simulink subsystem "VDBSCAN"  (R2022b)
settings: Solver=VariableStepAuto  StartTime=0.0  StopTime=10.0  RelTol=1e-3
settings Model: Creator=smryk  LastModifiedBy=sathu

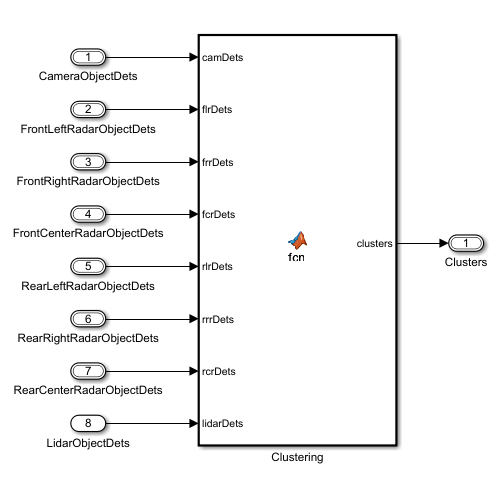
[thumbnail: Simulink's stored preview of the top-level diagram]
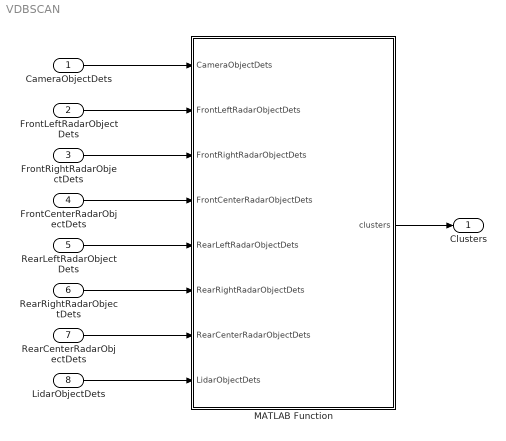
== system VDBSCAN ==
  CameraObjectDets : Inport  OutDataTypeStr=Bus: BusObjectDetections1
  FrontLeftRadarObjectDets : Inport  Port=2  OutDataTypeStr=Bus: BusDrivingRadarDataGenerator1
  FrontRightRadarObjectDets : Inport  Port=3  OutDataTypeStr=Bus: BusDrivingRadarDataGenerator1
  FrontCenterRadarObjectDets : Inport  Port=4  OutDataTypeStr=Bus: BusDrivingRadarDataGenerator1
  RearLeftRadarObjectDets : Inport  Port=5  OutDataTypeStr=Bus: BusDrivingRadarDataGenerator1
  RearRightRadarObjectDets : Inport  Port=6  OutDataTypeStr=Bus: BusDrivingRadarDataGenerator1
  RearCenterRadarObjectDets : Inport  Port=7  OutDataTypeStr=Bus: BusDrivingRadarDataGenerator1
  LidarObjectDets : Inport  Port=8
  MATLAB Function : MATLAB Function  TreatAsAtomicUnit=on
  Clusters : Outport  OutDataTypeStr=Bus: BusObjectDetections1
  wires:
  LidarObjectDets/1 -> MATLAB Function/8(LidarObjectDets)
  RearCenterRadarObjectDets/1 -> MATLAB Function/7(RearCenterRadarObjectDets)
  RearRightRadarObjectDets/1 -> MATLAB Function/6(RearRightRadarObjectDets)
  RearLeftRadarObjectDets/1 -> MATLAB Function/5(RearLeftRadarObjectDets)
  FrontCenterRadarObjectDets/1 -> MATLAB Function/4(FrontCenterRadarObjectDets)
  FrontRightRadarObjectDets/1 -> MATLAB Function/3(FrontRightRadarObjectDets)
  FrontLeftRadarObjectDets/1 -> MATLAB Function/2(FrontLeftRadarObjectDets)
  MATLAB Function/1(clusters) -> Clusters/1
  CameraObjectDets/1 -> MATLAB Function/1(CameraObjectDets)

== matlab function VDBSCAN/MATLAB Function ==
  data: CameraObjectDets input; clusters output Bus: BusObjectDetections1; FrontLeftRadarObjectDets input; FrontRightRadarObjectDets input; FrontCenterRadarObjectDets input; RearLeftRadarObjectDets input; RearRightRadarObjectDets input; RearCenterRadarObjectDets input; LidarObjectDets input
function clusters = fcn(CameraObjectDets, FrontLeftRadarObjectDets, FrontRightRadarObjectDets, FrontCenterRadarObjectDets, RearLeftRadarObjectDets, RearRightRadarObjectDets, RearCenterRadarObjectDets, LidarObjectDets)
    %clusters.Detections.Measurements(1)= xPos
    %clusters.Detections.Measurements(2)= yPos
    %clusters.NumDetections = number of clusters

    %format the data from the sensors
    sensorsData = formatSensorData(CameraObjectDets, FrontLeftRadarObjectDets, FrontRightRadarObjectDets, FrontCenterRadarObjectDets, RearLeftRadarObjectDets, RearRightRadarObjectDets, RearCenterRadarObjectDets, LidarObjectDets);
    
    k = 5; %NOTE: K can be adjusted 
    minPoints = k - 1; %minus one because k used in calculating epsilon has the points itself included as neighbouring points
    minDetections = 3; %minimum number of detections to validate a cluster

    epsilon = kNeighbours(sensorsData, k);

    %run DBSCAN
    allClusters = [0 0 0];
    for j = 1:size(epsilon, 1)
        idx = DBSCAN(epsilon(j), minPoints, sensorsData);

        clusterData = sensorsData(idx ~= -1, :);
        sensorsData = sensorsData(idx == -1, :);
        
        %Get the tracks 
        validIdx = idx(idx ~= -1);
        clusterNum = unique(validIdx);

        for m = 1:size(clusterNum,1)
            cluster = clusterData(validIdx == m, :);
            if (size(cluster,1) >= minDetections)
                centroid = mean(cluster);
                tracks = [centroid(1) centroid(2) size(cluster,1)];

                allClusters = [allClusters; tracks];
            end
        end  
    end
     
    finalClusters = allClusters(2:end,:); %strip off the first element since that was just a place hold for the size allTracks
    %finalClusters = [xPos yPos numDetections]

    measurements = zeros(50, 2);
    for j = 1:size(finalClusters, 1)
        measurements(j,:) = finalClusters(j,1:2);
    end
    

    clusters.NumDetections = size(finalClusters, 1);
    clusters.IsValidTime = boolean(0);
    
    fakeMeasurementParams.Frame = drivingCoordinateFrameType(0);
    fakeMeasurementParams.OriginPosition = [0; 0; 0];
    fakeMeasurementParams.Orientation = [0 0 0; 0 0 0; 0 0 0];
    fakeMeasurementParams.HasVelocity = boolean(0);
    
    fakeObjAttributes.TargetIndex = 0;

    for i = 1:50
        fakeDetection.Time = 0;
        fakeDetection.Measurement = [measurements(i,1); measurements(i,2); 0; 0; 0; 0];
        fakeDetection.MeasurementNoise = [0 0 0 0 0 0; 0 0 0 0 0 0; 0 0 0 0 0 0; 0 0 0 0 0 0; 0 0 0 0 0 0; 0 0 0 0 0 0];
        fakeDetection.SensorIndex = 0;
        fakeDetection.ObjectClassID = 0;
        fakeDetection.MeasurementParameters = fakeMeasurementParams;
        fakeDetection.ObjectAttributes = fakeObjAttributes;

        clusters.Detections(i) = fakeDetection;
    end
end 

function sensorsData = formatSensorData(CameraObjectDets, FrontLeftRadarObjectDets, FrontRightRadarObjectDets, FrontCenterRadarObjectDets, RearLeftRadarObjectDets, RearRightRadarObjectDets, RearCenterRadarObjectDets, LidarObjectDets)
    %% Format Sensor Data
    numFrontCamDets = CameraObjectDets.NumDetections;
    frontCamDetsArray = CameraObjectDets.Detections;
    
    numFrontLeftRadarDets = FrontLeftRadarObjectDets.NumDetections;
    frontLeftRadarDetsArray = FrontLeftRadarObjectDets.Detections;
    
    numFrontRightRadarDets = FrontRightRadarObjectDets.NumDetections;
    frontRightRadarDetsArray = FrontRightRadarObjectDets.Detections;


    numFrontCenterRadarDets = FrontCenterRadarObjectDets.NumDetections;
    frontCenterRadarDetsArray = FrontCenterRadarObjectDets.Detections;

    numRearLeftRadarDets = RearLeftRadarObjectDets.NumDetections;
    rearLeftRadarDetsArray = RearLeftRadarObjectDets.Detections;
    
    numRearRightRadarDets = RearRightRadarObjectDets.NumDetections;
    rearRightRadarDetsArray = RearRightRadarObjectDets.Detections;

    numRearCenterRadarDets = RearCenterRadarObjectDets.NumDetections;
    rearCenterRadarDetsArray = RearCenterRadarObjectDets.Detections;

    numLidarDets = LidarObjectDets.NumDetections;
    lidarObjectDetsArray = LidarObjectDets.Detections;
    
    %Get Front camera data [xPos, yPos]
    frontCamera = zeros(numFrontCamDets,2);
    for i = 1:numFrontCamDets
        detection = frontCamDetsArray(i);
        disp("Camera")
        disp(detection.MeasurementNoise)
        detectionState = detection.Measurement; 
        frontCamera(i,:)=[detectionState(1), detectionState(2)];
    end

    %Get front left radar data [xPos, yPos]
    frontLeftRadar = zeros(numFrontLeftRadarDets,2);
    for i = 1:numFrontLeftRadarDets
        detection = frontLeftRadarDetsArray(i);
        disp("Radar")
        disp(detection.MeasurementNoise)
        detectionState = detection.Measurement; 
        frontLeftRadar(i,:) = [detectionState(1), detectionState(2)];
    end

    %Get front right radar data [xPos, yPos]
    frontRightRadar = zeros(numFrontRightRadarDets, 2);
    for i = 1:numFrontRightRadarDets
        detection = frontRightRadarDetsArray(i);
        detectionState = detection.Measurement; 
        frontRightRadar(i,:) = [detectionState(1), detectionState(2)];
    end

    %Get front center radar data [xPos, yPos]
    frontCenterRadar = zeros(numFrontCenterRadarDets, 2);
    for i = 1:numFrontCenterRadarDets
        detection = frontCenterRadarDetsArray(i);
        detectionState = detection.Measurement; 
        frontCenterRadar(i,:) = [detectionState(1), detectionState(2)];
    end

    %Get rear left radar data [xPos, yPos]
    rearLeftRadar = zeros(numRearLeftRadarDets,2);
    for i = 1:numRearLeftRadarDets
        detection = rearLeftRadarDetsArray(i);
        detectionState = detection.Measurement; 
        rearLeftRadar(i,:) = [detectionState(1), detectionState(2)];
    end

    %Get rear right radar data [xPos, yPos]
    rearRightRadar = zeros(numRearRightRadarDets, 2);
    for i = 1:numRearRightRadarDets
        detection = rearRightRadarDetsArray(i);
        detectionState = detection.Measurement; 
        rearRightRadar(i,:) = [detectionState(1), detectionState(2)];
    end

    %Get rear center radar data [xPos, yPos]
    rearCenterRadar = zeros(numRearCenterRadarDets, 2);
    for i = 1:numRearCenterRadarDets
        detection = rearCenterRadarDetsArray(i);
        detectionState = detection.Measurement; 
        rearCenterRadar(i,:) = [detectionState(1), detectionState(2)];
    end

    %Get lidar data [xPos, yPos]
    lidar = zeros(numLidarDets,2);
    for i = 1:numLidarDets
        detection = lidarObjectDetsArray(i);
        detectionState = detection.Measurement; 
        lidar(i,:)=[detectionState(1), detectionState(2)];
    end

    %combine sensors' data into one matrix 
    sensorsData = [frontCamera; frontLeftRadar; frontRightRadar; frontCenterRadar; rearLeftRadar; rearRightRadar; rearCenterRadar; lidar];
end

function epsilon = kNeighbours(sensorsData, k)
    %INPUT
    %sensorsData = [xPos yPos]
    %k = int
    %OUTPUT
    %epsilon = [radius]
  
    kPoints = zeros(size(sensorsData,1),1);
    %find the kth nearest neighbour of all data points
    for i = 1:size(sensorsData, 1)
        currentPoint = sensorsData(i,:);
        distance = sqrt((sensorsData(:,1) - currentPoint(1)).^2 + (sensorsData(:,2) - currentPoint(2)).^2);
        sortedDistance = sort(distance);
        kPoints(i) = sortedDistance(k);
    end

    kPoints = sort(kPoints);
    [~, similarPoints] = ischange(kPoints);
    epsilon = unique(similarPoints);
    epsilon = epsilon(epsilon <= 1.5); %only allow epsilons less than 1.5

end

function clusters = DBSCAN(radius, minPoints, sensorsData)
    %% Algorithm- DBSCAN
    %INPUT
    %radius = int
    %minPoints = int
    %sensorsData = [xPos yPos] 
    %OUTPUT
    %clusters = [clusterNum] 
    
    %Find Core Points
    dataDim = size(sensorsData, 1);
    pointTypeData = [sensorsData zeros(dataDim,1)]; %[xPos yPos isCorePoint]

    for i = 1: dataDim
        pointTypeData(i,3) = findCorePoint(sensorsData(i,:), sensorsData, radius, minPoints);
    end

    %Organize the Corepoints into clusters
    corePointClusters = groupCorePoints(pointTypeData, radius);

    %Classify border points into the clusters
    clusterData = classifyBorderPoints(pointTypeData, corePointClusters, radius);

    clusters = clusterData(:,4);
end

%Determines if a point is a Core Point
function isCorePoint = findCorePoint (currentPoint, sensorData, radius, minPoints)
    %INPUT
    % currentPoint = [xPos yPos]
    %sensorData = [xPos yPos]
    %radius = float
    %minPoint = int
    %OUTPUT
    %isCorePoint = Boolean

    %find the relative distance of all points in the Data to the current point
    relativeDistance = sqrt((sensorData(:,1) - currentPoint(1)).^2 + (sensorData(:,2) - currentPoint(2)).^2);

    %Check if the number of neghboring points is less than minPoints
    counter = 0;
    for i = 1:size(sensorData,1)
        if (relativeDistance(i) <= radius)
            counter = counter + 1;
            if (counter >= minPoints)
                isCorePoint = true;
                return;
            end
        end
    end
    isCorePoint = false;
end

%Group core points into clusters
function corePointClusters = groupCorePoints(pointTypeData, radius)
    %INPUT
    %pointTypeData = [Boolean]
    %radius = float 
    %OUTPUT
    %corePointClusters = [xPos yPos isCorePoint clusterNum]
    
    corePointClusters = [pointTypeData ones(size(pointTypeData,1),1).*-1 ]; %[xPos yPos isCorePoint clusterNum]
    corePointData = [pointTypeData(pointTypeData(:,3) == 1, 1:2) find(pointTypeData(:,3) == 1)]; %[xPos yPos index] for Core Points in corePointCluster, index refers to location of point in corePointCluster
    cluster = []; %[xPos, yPos, clusterNum]
    clusterNumber = 1;

    while size(corePointData, 1) ~= 0
        %Takes whatever is first in corePointData as starting point for cluster
        cluster = [corePointData(1,1:2) clusterNumber]; %[xPos yPos clusterNum]
        
        %update the status of that point to the current cluster num
        corePointClusters(corePointData(1,3),4) = clusterNumber;

        corePointData = corePointData(2:end, :); %remove the point from the dataset so we don't have duplicates
        counter = 1;

        while counter <= size(cluster,1)
            %Use the position counter of cluster as a pointer to compare neighbouring core points
            %Use the first two columns of cluster as it contains the xPos and yPos
            currentPoint = cluster(counter,1:2);
           
            %Find the relative position of all remaining corePoints to the current point
            relativeDistance = sqrt((corePointData(:,1) - currentPoint(1)).^2 + (corePointData(:,2) - currentPoint(2)).^2);
        
            %Find the locations of neighbouring points in the data 
            neighbouringPointsLoc = relativeDistance <= radius;
        
            %Update cluster with new core points
            newCorePoints = corePointData(neighbouringPointsLoc, 1:2);
            newPoints = [newCorePoints ones(size(newCorePoints,1),1)*clusterNumber]; %[xPos, yPos, clusterNum]
            cluster = [cluster; newPoints];
        
            %update the clusterNum of the points based on their locations
            corePointClusters(corePointData(neighbouringPointsLoc,3),4) = clusterNumber;

            %Delete the classified core points from the temporary dataset
            corePointData(neighbouringPointsLoc, :) = [];
    
            counter = counter + 1;
        end
        %increase cluster number
        clusterNumber = clusterNumber + 1;
    end 
end

%Classifies border points into clusters
function clusterData = classifyBorderPoints(pointTypeData, clusterData, radius)
    %INPUT
    %pointTypeData = [Boolean]
    %clusterData = [xPos yPos isCorePoint clusterNum]
    %radius = int
    %OUTPUT
    %clusterData = [xPos yPos isCorePoint clusterNum]
    
    %Loop through each non Core Point
    nonCorePointData = [pointTypeData(pointTypeData(:,3) == 0, 1:2) find(pointTypeData(:,3) == 0)];

    for i = 1 : size(nonCorePointData, 1)
        currentPoint = nonCorePointData(i, :);

        for j = 1 : size(clusterData, 1)
            %Calculate the distance between the core point and the current point
            corePoint = clusterData(j,1:2);
            relativeDistance1D = sqrt((corePoint(1) - currentPoint(1)).^2 + (corePoint(2) - currentPoint(2)).^2);
        
            %Determine if current point is close enough to core point to be
            %part of the core point's cluster
            if relativeDistance1D <= radius
                clusterNumber = clusterData(j,4);
                clusterData(currentPoint(3),4) = clusterNumber;
                break
            end
        end
    end
end
